simulink model "foc_ctrl"  (R2023b)
settings: Solver=VariableStepAuto  StartTime=0.0  StopTime=10.0  RelTol=1e-3
settings Model: Creator=94570  LastModifiedBy=94570

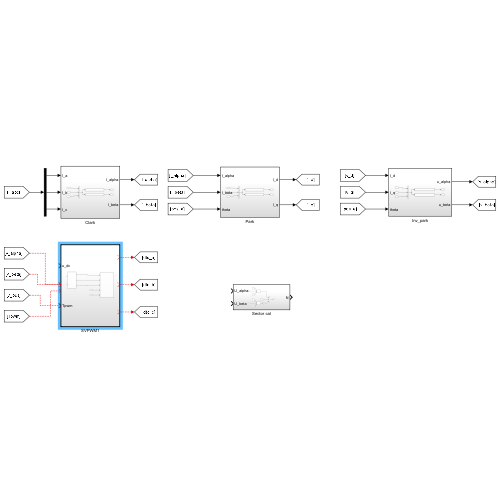
[thumbnail: Simulink's stored preview of the top-level diagram]
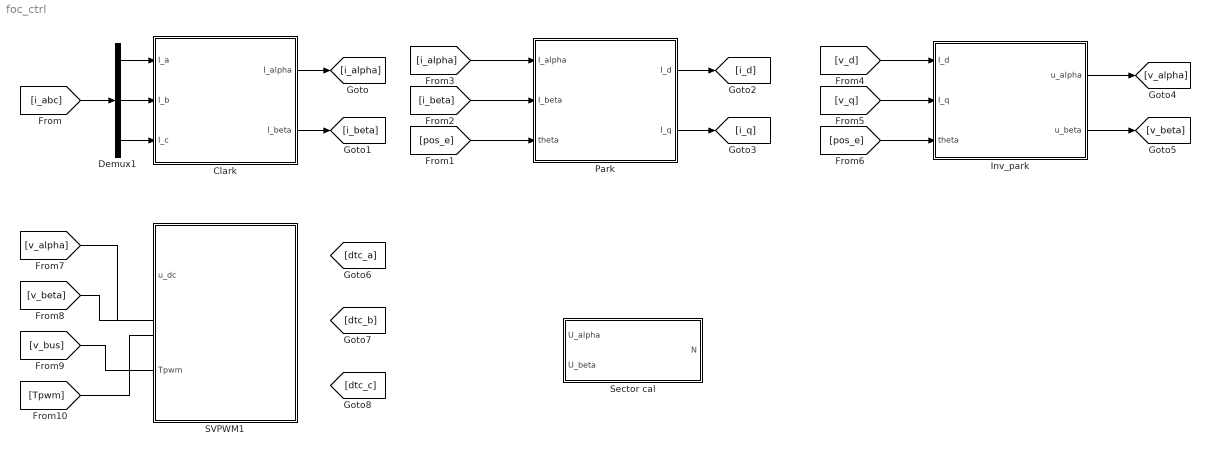
== system foc_ctrl ==
  Clark : Subsystem
  Demux1 : Demux  Outputs=3
  Inv_park : Subsystem
  Park : Subsystem
  SVPWM1 : Subsystem  TreatAsAtomicUnit=on
      settings: RTWSystemCode=Nonreusable function  RTWFcnNameOpts=Use subsystem name
  Sector cal : Subsystem
  wires:
  [i_abc] -> Demux1/1
  Demux1/2 -> Clark/2(I_b)
  Demux1/1 -> Clark/1(I_a)
  Demux1/3 -> Clark/3(I_c)
  Clark/1(I_alpha) -> [i_alpha]
  Clark/2(I_beta) -> [i_beta]
  [pos_e] -> Park/3(theta)
  [i_alpha] -> Park/1(I_alpha)
  [i_beta] -> Park/2(I_beta)
  Park/1(I_d) -> [i_d]
  Park/2(I_q) -> [i_q]
  [v_d] -> Inv_park/1(I_d)
  [pos_e] -> Inv_park/3(theta)
  [v_q] -> Inv_park/2(I_q)
  Inv_park/1(u_alpha) -> [v_alpha]
  Inv_park/2(u_beta) -> [v_beta]
  [v_alpha] -> ?
  [v_bus] -> ?
  [v_beta] -> ?
  [Tpwm] -> ?
  ? -> [dtc_a]
  ? -> [dtc_b]
  ? -> [dtc_c]

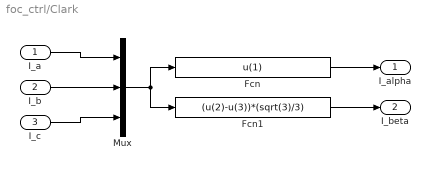
== system foc_ctrl/Clark ==
  I_a : Inport
  I_b : Inport  Port=2
  I_c : Inport  Port=3
  Fcn : Fcn  Expr=u(1)
  Fcn1 : Fcn  Expr=(u(2)-u(3))*(sqrt(3)/3)
  Mux : Mux  Inputs=3
  I_alpha : Outport
  I_beta : Outport  Port=2
  wires:
  I_a/1 -> Mux/1
  I_b/1 -> Mux/2
  I_c/1 -> Mux/3
  Mux/1 -> Fcn1/1, Fcn/1
  Fcn/1 -> I_alpha/1
  Fcn1/1 -> I_beta/1

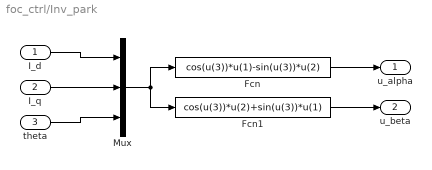
== system foc_ctrl/Inv_park ==
  I_d : Inport
  I_q : Inport  Port=2
  theta : Inport  Port=3
  Fcn : Fcn  Expr=cos(u(3))*u(1)-sin(u(3))*u(2)
  Fcn1 : Fcn  Expr=cos(u(3))*u(2)+sin(u(3))*u(1)
  Mux : Mux  Inputs=3
  u_alpha : Outport
  u_beta : Outport  Port=2
  wires:
  theta/1 -> Mux/3
  I_q/1 -> Mux/2
  I_d/1 -> Mux/1
  Fcn/1 -> u_alpha/1
  Mux/1 -> Fcn1/1, Fcn/1
  Fcn1/1 -> u_beta/1

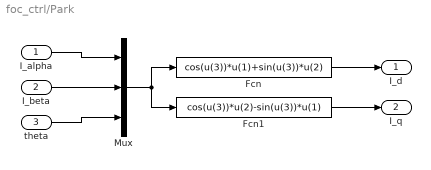
== system foc_ctrl/Park ==
  I_alpha : Inport
  I_beta : Inport  Port=2
  theta : Inport  Port=3
  Fcn : Fcn  Expr=cos(u(3))*u(1)+sin(u(3))*u(2)
  Fcn1 : Fcn  Expr=cos(u(3))*u(2)-sin(u(3))*u(1)
  Mux : Mux  Inputs=3
  I_d : Outport
  I_q : Outport  Port=2
  wires:
  I_alpha/1 -> Mux/1
  I_beta/1 -> Mux/2
  theta/1 -> Mux/3
  Mux/1 -> Fcn1/1, Fcn/1
  Fcn/1 -> I_d/1
  Fcn1/1 -> I_q/1

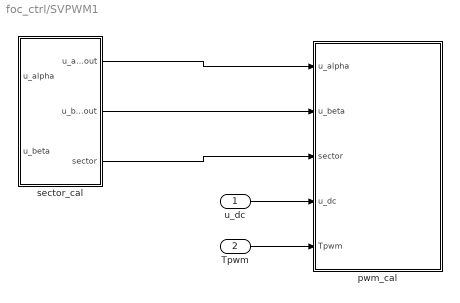
== system foc_ctrl/SVPWM1 ==
  u_dc : Inport
  Tpwm : Inport  Port=2
  pwm_cal : Subsystem
  sector_cal : Subsystem
  wires:
  u_dc/1 -> pwm_cal/4(u_dc)
  Tpwm/1 -> pwm_cal/5(Tpwm)
  sector_cal/3(sector) -> pwm_cal/3(sector)
  sector_cal/2(u_beta_out) -> pwm_cal/2(u_beta)
  sector_cal/1(u_alpha_out) -> pwm_cal/1(u_alpha)

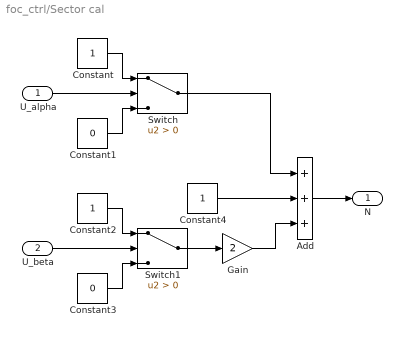
== system foc_ctrl/Sector cal ==
  U_alpha : Inport
  U_beta : Inport  Port=2
  Add : Sum  Inputs=+++
  Constant : Constant
  Constant1 : Constant  Value=0
  Constant2 : Constant
  Constant3 : Constant  Value=0
  Constant4 : Constant
  Gain : Gain  Gain=2
  Switch : Switch  Criteria=u2 > Threshold  SaturateOnIntegerOverflow=off  InputSameDT=off
  Switch1 : Switch  Criteria=u2 > Threshold  SaturateOnIntegerOverflow=off  InputSameDT=off
  N : Outport
  wires:
  U_alpha/1 -> Switch/2
  Constant/1 -> Switch/1
  Constant1/1 -> Switch/3
  Constant2/1 -> Switch1/1
  U_beta/1 -> Switch1/2
  Constant3/1 -> Switch1/3
  Switch1/1 -> Gain/1
  Gain/1 -> Add/3
  Switch/1 -> Add/1
  Constant4/1 -> Add/2
  Add/1 -> N/1

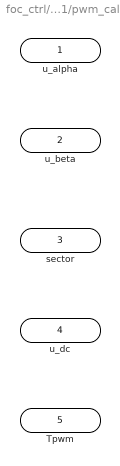
== system foc_ctrl/SVPWM1/pwm_cal ==
  u_alpha : Inport
  u_beta : Inport  Port=2
  sector : Inport  Port=3
  u_dc : Inport  Port=4
  Tpwm : Inport  Port=5

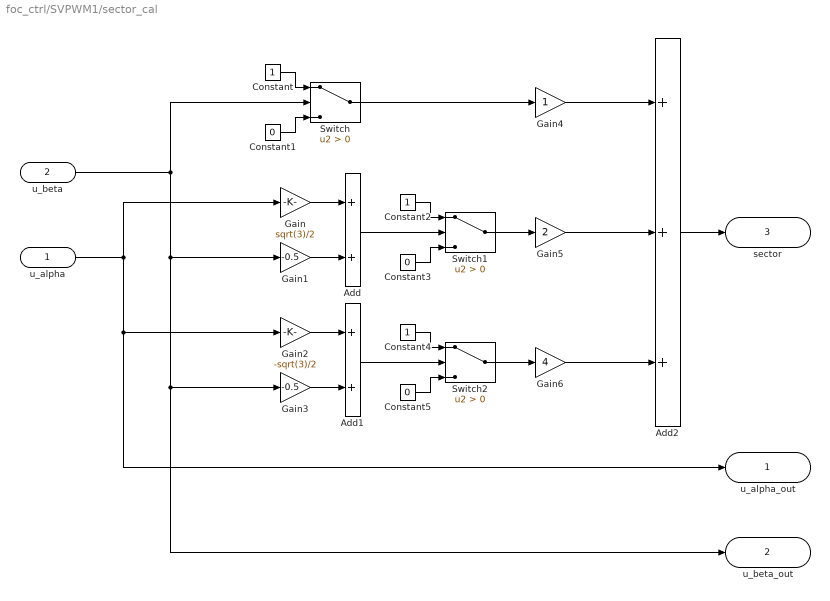
== system foc_ctrl/SVPWM1/sector_cal ==
  u_alpha : Inport
  u_beta : Inport  Port=2
  Add : Sum
  Add1 : Sum
  Add2 : Sum  Inputs=+++
  Constant : Constant
  Constant1 : Constant  Value=0
  Constant2 : Constant
  Constant3 : Constant  Value=0
  Constant4 : Constant
  Constant5 : Constant  Value=0
  Gain : Gain  Gain=sqrt(3)/2
  Gain1 : Gain  Gain=-0.5
  Gain2 : Gain  Gain=-sqrt(3)/2
  Gain3 : Gain  Gain=-0.5
  Gain4 : Gain
  Gain5 : Gain  Gain=2
  Gain6 : Gain  Gain=4
  Switch : Switch  Criteria=u2 > Threshold  SaturateOnIntegerOverflow=off  InputSameDT=off
  Switch1 : Switch  Criteria=u2 > Threshold  SaturateOnIntegerOverflow=off  InputSameDT=off
  Switch2 : Switch  Criteria=u2 > Threshold  SaturateOnIntegerOverflow=off  InputSameDT=off
  u_alpha_out : Outport
  u_beta_out : Outport  Port=2
  sector : Outport  Port=3
  wires:
  Add/1 -> Switch1/2
  Constant3/1 -> Switch1/3
  Constant2/1 -> Switch1/1
  Constant/1 -> Switch/1
  Constant5/1 -> Switch2/3
  Gain1/1 -> Add/2
  Add1/1 -> Switch2/2
  Gain4/1 -> Add2/1
  Gain/1 -> Add/1
  Switch2/1 -> Gain6/1
  Switch/1 -> Gain4/1
  Gain6/1 -> Add2/3
  u_beta/1 -> Gain1/1, u_beta_out/1, Gain3/1, Switch/2
  u_alpha/1 -> Gain/1, u_alpha_out/1, Gain2/1
  Gain3/1 -> Add1/2
  Gain2/1 -> Add1/1
  Constant4/1 -> Switch2/1
  Gain5/1 -> Add2/2
  Constant1/1 -> Switch/3
  Switch1/1 -> Gain5/1
  Add2/1 -> sector/1
